simulink model "Charging_CCCV"  (R2016a)
settings: Solver=VariableStepAuto  StartTime=0.0  StopTime=5000  RelTol=1e-3
undefined symbols (not defined in the file): Ion, Lithium
libraries: powerlib x5, electricdrivelib x1
settings Model: Creator=a7med  LastModifiedBy=a7med

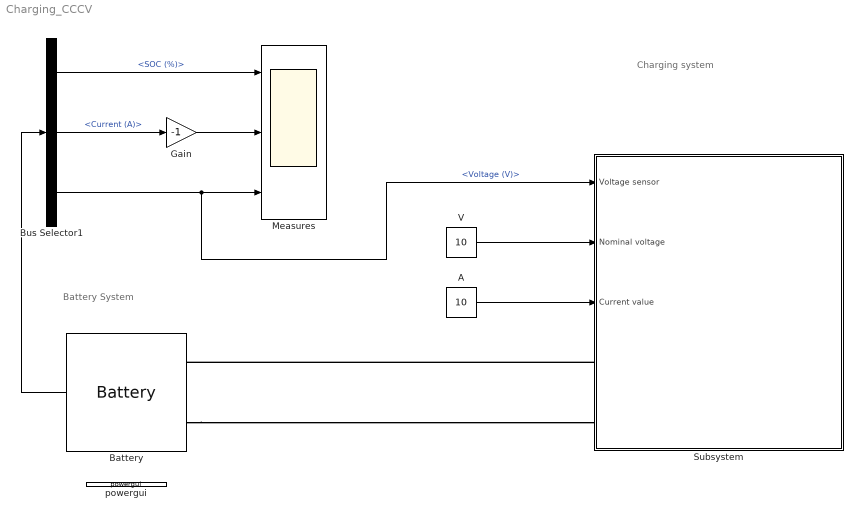
== system Charging_CCCV ==
  note: Battery System
  note: Charging system
  A : Constant  Value=10
  Battery : electricdrivelib/Extra Sources/Battery  BatType=Lithium-Ion  ShowTempParam=off  ThermalPreset=no  NomV=9  NomQ=6.5  SOC=0  Batt_Tr=30  PresetModel=on  MaxQ=6.5  MinV=6.75  FullV=10.4759  Dis_rate=2.8261  R=0.013846  Normal_OP=5.8783  expZone="[9.7235     0.31935]"  current=[6.5 13 32.5]  Units=Time  Tci=25  NomT=25  T2=0  MaxQ2=2.208  FullV2=3.45  Normal_OP2=2.8  expZone2="[3.22        0.23]"  Rca=0.6  ti=1000  Dp=0
  Bus Selector1 : BusSelector  OutputSignals=SOC (%),Current (A),Voltage (V)
  Gain : Gain  Gain=-1
  "Measures " : Scope  NumInputPorts=3
  Subsystem : Subsystem
      settings: AttributesFormatString=CCCV charging system
  V : Constant  Value=10
  powergui : powerlib/powergui  SimulationMode=Continuous  SolverType=Tustin  SampleTime=0.001  frequency=60  SPID=on  DisableSnubberDevices=off  DisableRonSwitches=off  DisableVfSwitches=off  SwTol=0  DisplayEquations=off  Interpol=off  ExternalGateDelay=off  methode=off  Ts=0  FunctionMessages=off  echomessages=off  HookPort=off  EnableUseOfTLC=off  x0status=blocks  frequencyindice=0  Pbase=100e6  ErrMax=1e-4  Iterations=50  UnitsV=kV  UnitsW=MW  buscounter=0  RestoreLinks=warning  ResistiveCurrentMeasurement=off  Frange=[0:2:500]  Ylog=off  Xlog=on  ShowGrid=off  save=off  variable=ZData  structure=0  ZoomFFT=on  StartTime=0.0  cycles=1  DisplayStyle=1  fundamental=60  FreqAxis=off  MaxFrequency=1000  frequencyindicesteady=1  RmsSteady=1  display=off
  wires:
  Battery/1 -> Bus Selector1/1
  Gain/1 -> "Measures "/2
  Bus Selector1/2 -> Gain/1  "<Current (A)>"
  V/1 -> Subsystem/2(Nominal voltage)
  A/1 -> Subsystem/3(Current value)
  Bus Selector1/1 -> "Measures "/1  "<SOC (%)>"
  Bus Selector1/3 -> Subsystem/1(Voltage sensor), "Measures "/3  "<Voltage (V)>"
  connections:
  Subsystem/LConn1 -- Battery/LConn1
  Battery/LConn2 -- Subsystem/LConn2

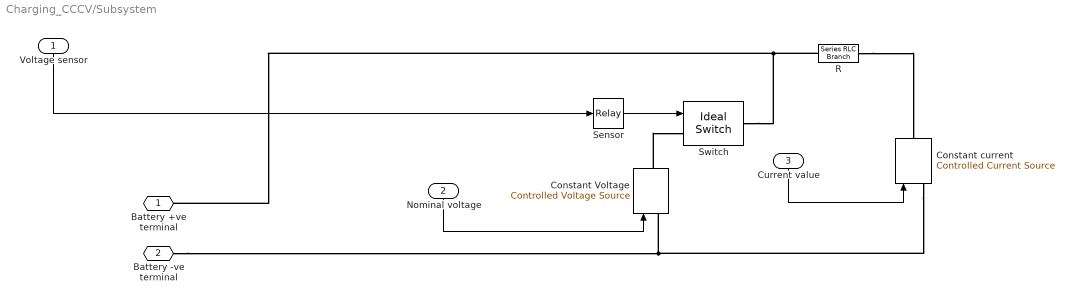
== system Charging_CCCV/Subsystem ==
  Voltage sensor : Inport
  Nominal voltage : Inport  Port=2
  Current value : Inport  Port=3
  Constant Voltage : powerlib/Electrical Sources/Controlled Voltage Source  Initialize=on  Source_Type=DC  Amplitude=0  Phase=0  Frequency=0  Measurements=None
  "Constant current " : powerlib/Electrical Sources/Controlled Current Source  Initialize=on  Source_Type=DC  Amplitude=0  Phase=0  Frequency=0  Measurements=None
  R : powerlib/Elements/Series RLC Branch  LConnTagsString=__new0  RConnTagsString=__new0  BranchType=R  Resistance=1000  Inductance=0  SetiL0=off  InitialCurrent=0  Capacitance=0  Setx0=off  InitialVoltage=0  Measurements=Branch voltage
  Sensor : Relay  OnSwitchValue=10  OffSwitchValue=10
  Switch : powerlib/Power Electronics/Ideal Switch  Ron=0  Lon=0  IC=0  Rs=1e5  Cs=inf  Measurements=off
  Battery +ve terminal : PMIOPort  Port=1  Side=Left
  "Battery -ve terminal " : PMIOPort  Port=2  Side=Left
  wires:
  Nominal voltage/1 -> Constant Voltage/1
  Current value/1 -> "Constant current "/1
  Sensor/1 -> Switch/1
  Voltage sensor/1 -> Sensor/1
  connections:
  "Constant current "/LConn1 -- "Battery -ve terminal "/RConn1 -- Constant Voltage/LConn1
  R/LConn1 -- Battery +ve terminal/RConn1 -- Switch/RConn1
  R/RConn1 -- "Constant current "/RConn1
  Constant Voltage/RConn1 -- Switch/LConn1
